simulink model "Offline_FLIP_FLOP_2019"  (R2019b)
settings: Solver=VariableStepAuto  StartTime=0.0  StopTime=50  RelTol=1e-3
values from neighbouring files (symbols this model uses):
  alpha_max = 15    [Flip_Flop_StartUp.m]
  theta_max = 45    [Flip_Flop_StartUp.m]
libraries: simulink x3, simulink_extras x1
settings Model: Creator=albif  LastModifiedBy=albif
settings DebuggingCC: UnconnectedInputMsg=none  UnconnectedOutputMsg=none  UnconnectedLineMsg=none  SFMachineParentedDataDiag=error
settings ModelReferenceCC: EnableRefExpFcnMdlSchedulingChecks=off
settings RTWCC: Description=Generic Real-Time Target

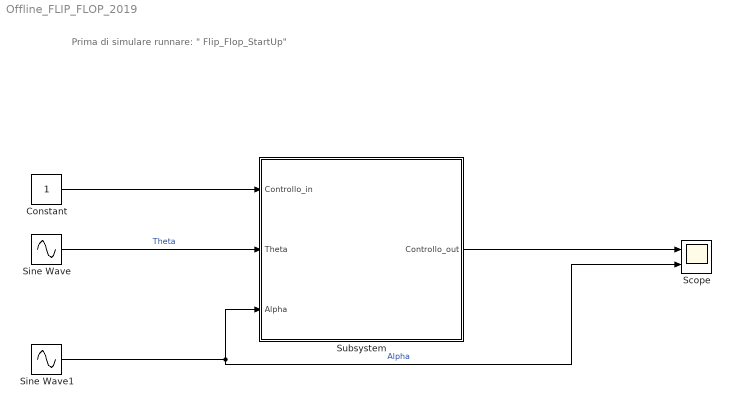
== system Offline_FLIP_FLOP_2019 ==
  note: Prima di simulare runnare: " Flip_Flop_StartUp"
  Constant : Constant
  Scope : Scope  NumInputPorts=2
  Sine Wave : Sin  Frequency=0.5  SampleTime=0
  Sine Wave1 : Sin  Amplitude=0.3  Frequency=0.3  Phase=pi/4  SampleTime=0
  Subsystem : Subsystem
  wires:
  Sine Wave1/1 -> Scope/2, Subsystem/3(Alpha)  "Alpha"
  Constant/1 -> Subsystem/1(Controllo_in)
  Subsystem/1(Controllo_out) -> Scope/1
  Sine Wave/1 -> Subsystem/2(Theta)  "Theta"

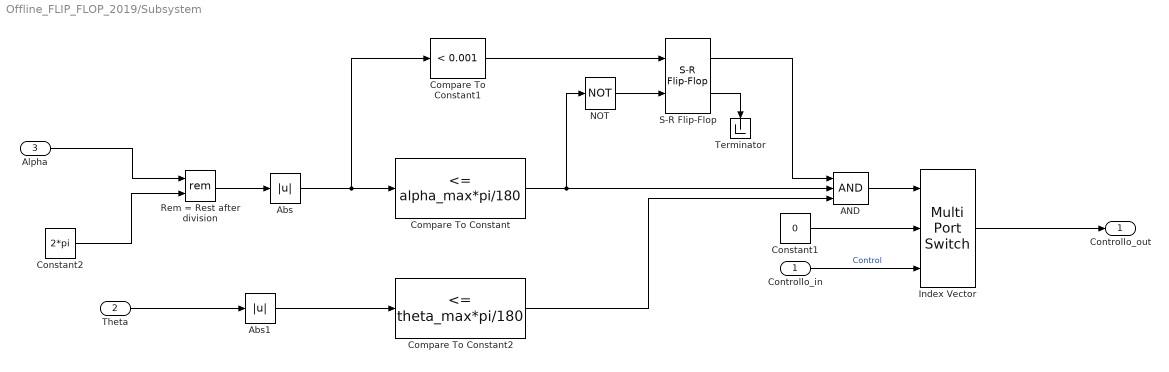
== system Offline_FLIP_FLOP_2019/Subsystem ==
  Controllo_in : Inport
  Theta : Inport  Port=2
  Alpha : Inport  Port=3
  AND : Logic  Inputs=3  IconShape=distinctive  AllPortsSameDT=off  OutDataTypeStr=boolean
  Abs : Abs
  Abs1 : Abs
  Compare To Constant : simulink/Logic and Bit Operations/Compare To Constant  relop=<=  const=alpha_max*pi/180  OutDataTypeStr=boolean
  Compare To Constant1 : simulink/Logic and Bit Operations/Compare To Constant  relop=<  const=0.001  OutDataTypeStr=boolean
  Compare To Constant2 : simulink/Logic and Bit Operations/Compare To Constant  relop=<=  const=theta_max*pi/180  OutDataTypeStr=boolean
  Constant1 : Constant  Value=0
  Constant2 : Constant  Value=2*pi
  Index Vector : MultiPortSwitch  DataPortOrder=Zero-based contiguous  Inputs=2  zeroidx=on
  NOT : Logic  Operator=NOT  IconShape=distinctive  AllPortsSameDT=off  OutDataTypeStr=boolean
  Rem = Rest after division : Math  Operator=rem  SignedPower=off  SaturateOnIntegerOverflow=on
  S-R Flip-Flop : simulink_extras/Flip Flops/S-R Flip-Flop  initial_condition=0
  Terminator : Terminator
  Controllo_out : Outport
  wires:
  NOT/1 -> S-R Flip-Flop/2
  Compare To Constant/1 -> AND/2, NOT/1
  Alpha/1 -> Rem = Rest after division/1
  Controllo_in/1 -> Index Vector/3  "Control"
  Constant1/1 -> Index Vector/2
  Rem = Rest after division/1 -> Abs/1
  S-R Flip-Flop/1 -> AND/1
  Constant2/1 -> Rem = Rest after division/2
  AND/1 -> Index Vector/1
  Abs/1 -> Compare To Constant/1, Compare To Constant1/1
  Compare To Constant1/1 -> S-R Flip-Flop/1
  Index Vector/1 -> Controllo_out/1
  S-R Flip-Flop/2 -> Terminator/1
  Theta/1 -> Abs1/1
  Abs1/1 -> Compare To Constant2/1
  Compare To Constant2/1 -> AND/3
